simulink subsystem "SocCorrection_SubSys"  (R2022b)
settings: Solver=VariableStepAuto  StartTime=0.0  StopTime=10.0  RelTol=1e-3
undefined symbols (not defined in the file): KeSoc_frc_SocMaxLim, KeSoc_frc_SocMinLim, KeSoc_nu_SocCorrnFac
settings Model: Creator=Niharika  LastModifiedBy=Niharika

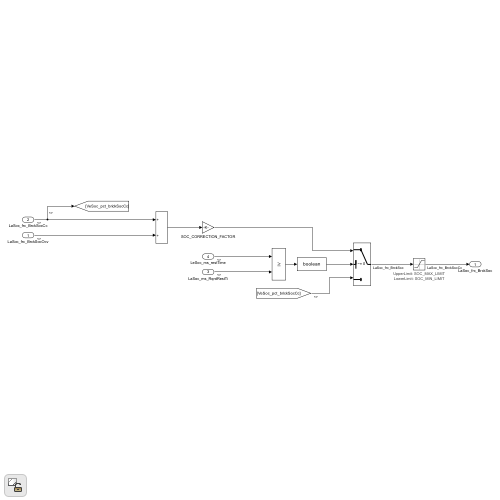
[thumbnail: Simulink's stored preview of the top-level diagram]
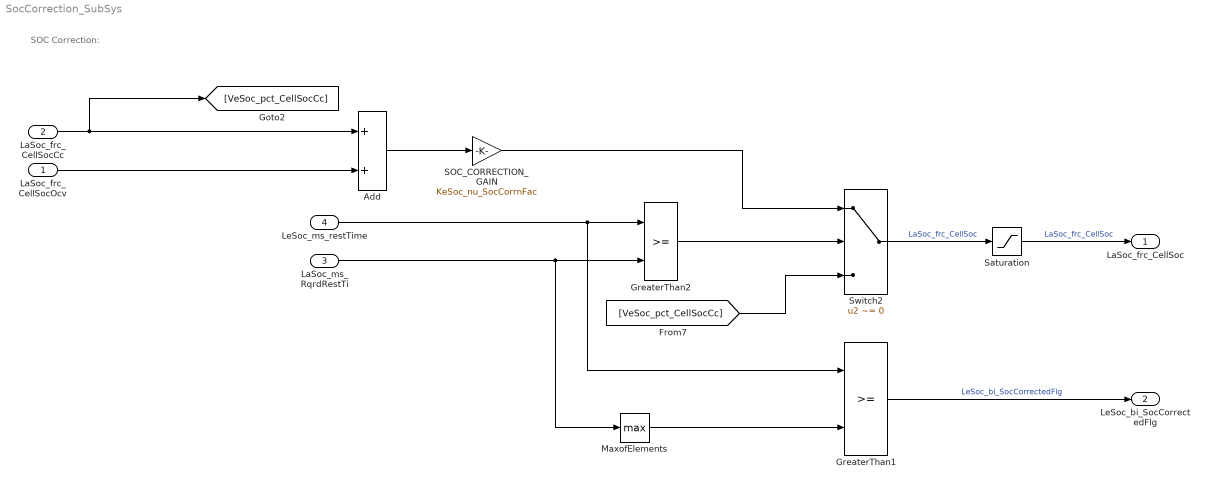
== system SocCorrection_SubSys ==
  note: SOC Correction:
  LaSoc_frc_CellSocOcv : Inport
  LaSoc_frc_CellSocCc : Inport  Port=2
  LaSoc_ms_RqrdRestTi : Inport  Port=3
  LeSoc_ms_restTime : Inport  Port=4
  Add : Sum
  GreaterThan1 : RelationalOperator  OutDataTypeStr=boolean  RndMeth=Simplest  InputSameDT=off
  GreaterThan2 : RelationalOperator  OutDataTypeStr=boolean  RndMeth=Simplest  InputSameDT=off
  MaxofElements : MinMax  Function=max
  SOC_CORRECTION_GAIN : Gain  Gain=KeSoc_nu_SocCorrnFac
  Saturation : Saturate  UpperLimit=KeSoc_frc_SocMaxLim  LowerLimit=KeSoc_frc_SocMinLim
      settings: AttributesFormatString=|
      | UpperLimit: %<UpperLimit>
      | LowerLimit: %<LowerLimit>
  Switch2 : Switch  Criteria=u2 ~= 0  SaturateOnIntegerOverflow=off  InputSameDT=off
  LaSoc_frc_CellSoc : Outport
  LeSoc_bi_SocCorrectedFlg : Outport  Port=2
  wires:
  Saturation/1 -> LaSoc_frc_CellSoc/1  "LaSoc_frc_CellSoc"
  Switch2/1 -> Saturation/1  "LaSoc_frc_CellSoc"
  SOC_CORRECTION_GAIN/1 -> Switch2/1
  LeSoc_ms_restTime/1 -> GreaterThan2/1, GreaterThan1/1
  LaSoc_frc_CellSocCc/1 -> Add/1, [VeSoc_pct_CellSocCc]
  GreaterThan2/1 -> Switch2/2
  [VeSoc_pct_CellSocCc] -> Switch2/3
  Add/1 -> SOC_CORRECTION_GAIN/1
  LaSoc_frc_CellSocOcv/1 -> Add/2
  GreaterThan1/1 -> LeSoc_bi_SocCorrectedFlg/1  "LeSoc_bi_SocCorrectedFlg"
  MaxofElements/1 -> GreaterThan1/2
  LaSoc_ms_RqrdRestTi/1 -> GreaterThan2/2, MaxofElements/1
